simulink model "LSTM_Acc"  (R2024b)
settings: Solver=FixedStepDiscrete  StartTime=0.0  StopTime=10.0  RelTol=1e-3
libraries: rtlinux_Library x11, simulink x2, deeplib x1
settings Model: Creator=petrc  LastModifiedBy=petrc
settings OptimizationCC: DefaultParameterBehavior=Inlined  EnhancedBackFolding=on  PassReuseOutputArgsAs=Individual arguments  ZeroExternalMemoryAtStartup=off  ZeroInternalMemoryAtStartup=off  OptimizeBlockOrder=speed  DifferentSizesBufferReuse=on  OptimizationCustomize=off  EfficientTunableParamExpr=on
settings DebuggingCC: ParameterTunabilityLossMsg=error
settings HardwareCC: ProdBitPerLong=64  ProdLargestAtomicInteger=LongLong  ProdLargestAtomicFloat=Double  ProdLongLongMode=on  ProdHWDeviceType=ARM Compatible->ARM Cortex-A (64-bit)
settings SFSimCC: MATLABDynamicMemAlloc=off
settings RTWCC: Description=Real-Time Linux (WSL/Yocto)  SystemTargetFile=rtlinux_ert.tlc  MakeCommand=make_rtw \  GenerateMakefile=off  TemplateMakefile=rtlinux_ert.tmf
settings CodeAppCC: ForceParamTrailComments=on  IgnoreCustomStorageClasses=off  OperatorAnnotations=on  SimulinkDataObjDesc=on  SFDataObjDesc=on  InsertBlockDesc=on
settings STFCustomTargetCC: TargetLibSuffix=.a  TargetLangStandard=C99 (ISO)  MultiwordLength=256  GenerateSampleERTMain=on  CombineOutputUpdateFcns=on  ERTCustomFileBanners=on  SupportContinuousTime=off  SupportNonInlinedSFcns=off  RemoveResetFunc=on  MATLABClassNameForMDSCustomization=Simulink.SoftwareTarget.ERTCustomization  ModelStepFunctionPrototypeControlCompliant=on  SystemTargetFile=rtlinux_ert.tlc
settings ERTTargetCC: TargetLangStandard=C99 (ISO)  GenerateSampleERTMain=on  ParMdlRefBuildCompliant=off  CompOptLevelCompliant=off  ConcurrentExecutionCompliant=off  CPPClassGenCompliant=off  UseToolchainInfoCompliant=off  ERTCustomFileTemplate=rtlinux_file_process.tlc

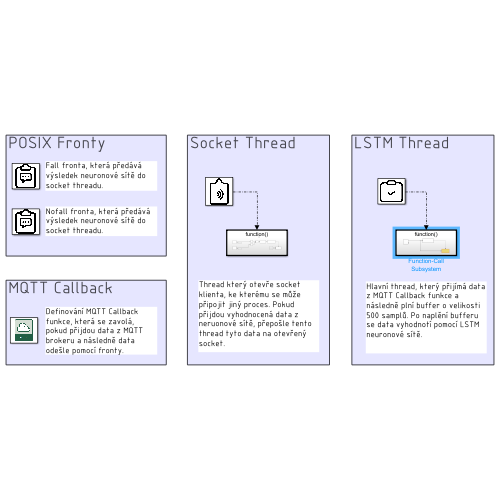
[thumbnail: Simulink's stored preview of the top-level diagram]
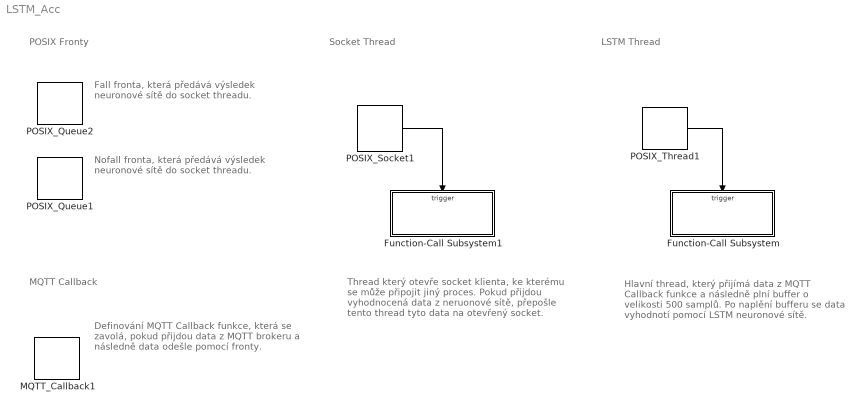
== system LSTM_Acc ==
  note: Nofall fronta, která předává výsledek neuronové sítě do socket threadu.
  note: Definování MQTT Callback funkce, která se zavolá, pokud přijdou data z MQTT brokeru a následně data odešle pomocí fronty.
  note: Socket Thread
  note: Thread který otevře socket klienta, ke kterému se může připojit jiný proces. Pokud přijdou vyhodnocená data z neruonové sítě, přepošle tento thread tyto data na otevřený socket.
  note: Fall fronta, která předává výsledek neuronové sítě do socket threadu.
  note: POSIX Fronty
  note: LSTM Thread
  note: Hlavní thread, který přijímá data z MQTT Callback funkce a následně plní buffer o velikosti 500 samplů. Po naplění bufferu se data vyhodnotí pomocí LSTM neuronové sítě.
  note: MQTT Callback
  Function-Call Subsystem : Subsystem  TreatAsAtomicUnit=on
  Function-Call Subsystem1 : Subsystem  TreatAsAtomicUnit=on
  MQTT_Callback1 : rtlinux_Library/MQTT_Callback  address=tcp://192.168.0.117:1883  clientid=CSubscriber  topic=/mpu6050/accel  qos=1  data_n=1  queue_name=accel_queue  length=10
      settings: SourceProductName=LINUX Library
  POSIX_Queue1 : rtlinux_Library/POSIX_Queue  QueueName=nofall_queue  QueueLenght=5
      settings: SourceProductName=LINUX Library
  POSIX_Queue2 : rtlinux_Library/POSIX_Queue  QueueName=fall_queue  QueueLenght=5
      settings: SourceProductName=LINUX Library
  POSIX_Socket1 : rtlinux_Library/POSIX_Socket  SocketName=/tmp/mysocket  Backlog=5  tickRes=10
      settings: SourceProductName=LINUX Library
  POSIX_Thread1 : rtlinux_Library/POSIX_Thread  TaskName=lstm_thread  TickRes=10  SchedPolicy=SCHED_OTHER  ThreadPriority=0  LockMemory=on  Affinity0=on  Affinity1=on  Affinity2=on  Affinity3=on
      settings: SourceProductName=LINUX Library
  wires:
  POSIX_Thread1/1 -> Function-Call Subsystem/Trigger
  POSIX_Socket1/1 -> Function-Call Subsystem1/Trigger

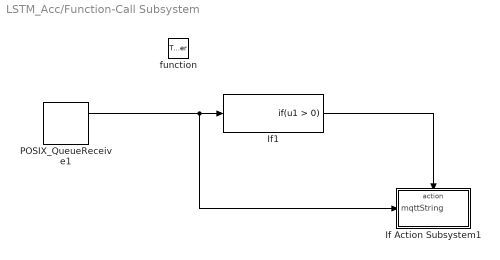
== system LSTM_Acc/Function-Call Subsystem ==
  function : TriggerPort  TriggerType=function-call  VariantControl=(inherit)
  If Action Subsystem1 : Subsystem  TreatAsAtomicUnit=on
  If1 : If  ShowElse=off
  POSIX_QueueReceive1 : rtlinux_Library/POSIX_QueueReceive  QueueName=accel_queue  buffer_enable=1  buffer_size=1024  buffer_name=receive_buffer
      settings: SourceProductName=LINUX Library
  wires:
  If1/1 -> If Action Subsystem1/Action
  POSIX_QueueReceive1/1 -> If Action Subsystem1/1(mqttString), If1/1

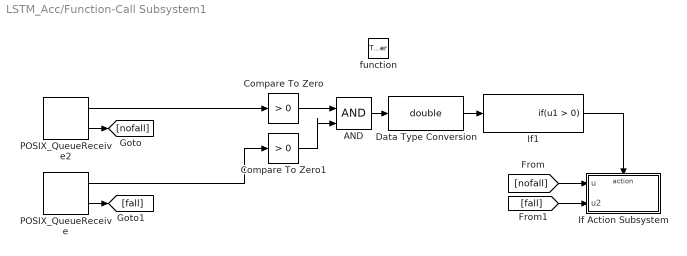
== system LSTM_Acc/Function-Call Subsystem1 ==
  function : TriggerPort  TriggerType=function-call  VariantControl=(inherit)
  AND : Logic  IconShape=distinctive  AllPortsSameDT=off  OutDataTypeStr=boolean
  Compare To Zero : simulink/Logic and Bit Operations/Compare To Zero  relop=>  OutDataTypeStr=boolean
  Compare To Zero1 : simulink/Logic and Bit Operations/Compare To Zero  relop=>  OutDataTypeStr=boolean
  Data Type Conversion : DataTypeConversion  OutDataTypeStr=double  SaturateOnIntegerOverflow=off  RndMeth=Floor
  If Action Subsystem : Subsystem  TreatAsAtomicUnit=on
  If1 : If  ShowElse=off
  POSIX_QueueReceive : rtlinux_Library/POSIX_QueueReceive  QueueName=fall_queue  buffer_enable=0  buffer_size=0  buffer_name=0
      settings: SourceProductName=LINUX Library
  POSIX_QueueReceive2 : rtlinux_Library/POSIX_QueueReceive  QueueName=nofall_queue  buffer_enable=0  buffer_size=0  buffer_name=0
      settings: SourceProductName=LINUX Library
  wires:
  POSIX_QueueReceive2/1 -> Compare To Zero/1
  POSIX_QueueReceive/1 -> Compare To Zero1/1
  If1/1 -> If Action Subsystem/Action
  POSIX_QueueReceive2/2 -> [nofall]
  POSIX_QueueReceive/2 -> [fall]
  [nofall] -> If Action Subsystem/1(u)
  [fall] -> If Action Subsystem/2(u2)
  Compare To Zero/1 -> AND/1
  Compare To Zero1/1 -> AND/2
  AND/1 -> Data Type Conversion/1
  Data Type Conversion/1 -> If1/1

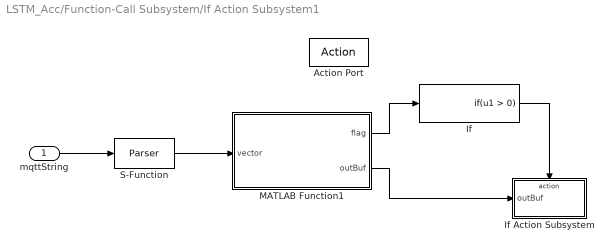
== system LSTM_Acc/Function-Call Subsystem/If Action Subsystem1 ==
  mqttString : Inport
  Action Port : ActionPort  ActionPortLabel=if(u1 > 0)
  If : If  ShowElse=off
  If Action Subsystem : Subsystem  TreatAsAtomicUnit=on
  MATLAB Function1 : MATLAB Function  TreatAsAtomicUnit=on
  S-Function : S-Function  FunctionName=Parser  SFunctionDeploymentMode=off  EnableBusSupport=off
  wires:
  If/1 -> If Action Subsystem/Action
  MATLAB Function1/1(flag) -> If/1
  MATLAB Function1/2(outBuf) -> If Action Subsystem/1(outBuf)
  mqttString/1 -> S-Function/1
  S-Function/1 -> MATLAB Function1/1(vector)

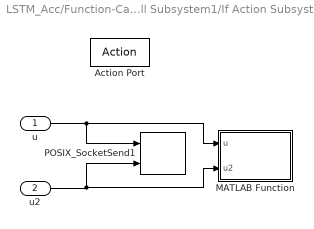
== system LSTM_Acc/Function-Call Subsystem1/If Action Subsystem ==
  u : Inport
  u2 : Inport  Port=2
  Action Port : ActionPort  ActionPortLabel=if(u1 > 0)
  MATLAB Function : MATLAB Function  TreatAsAtomicUnit=on
  POSIX_SocketSend1 : rtlinux_Library/POSIX_SocketSend  statement=%.3f %.3f  data_num=2
      settings: SourceProductName=LINUX Library
  wires:
  u/1 -> POSIX_SocketSend1/1, MATLAB Function/1(u)
  u2/1 -> POSIX_SocketSend1/2, MATLAB Function/2(u2)

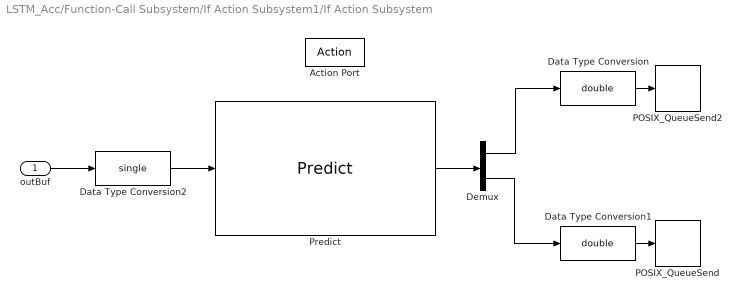
== system LSTM_Acc/Function-Call Subsystem/If Action Subsystem1/If Action Subsystem ==
  outBuf : Inport
  Action Port : ActionPort  ActionPortLabel=if(u1 > 0)
  Data Type Conversion : DataTypeConversion  OutDataTypeStr=double  SaturateOnIntegerOverflow=off  RndMeth=Floor
  Data Type Conversion1 : DataTypeConversion  OutDataTypeStr=double  SaturateOnIntegerOverflow=off  RndMeth=Floor
  Data Type Conversion2 : DataTypeConversion  OutDataTypeStr=single  SaturateOnIntegerOverflow=off  RndMeth=Floor
  Demux : Demux  Outputs=2
  POSIX_QueueSend : rtlinux_Library/POSIX_QueueSend  QueueName=fall_queue
      settings: SourceProductName=LINUX Library
  POSIX_QueueSend2 : rtlinux_Library/POSIX_QueueSend  QueueName=nofall_queue
      settings: SourceProductName=LINUX Library
  Predict : deeplib/Predict  Network=Network from MAT-file  NetworkFunction=squeezenet  NetworkFilePath=C:\Users\petrc\MATLAB\rtlinux_ert\Examples\LSTM_Acc\net.mat  MiniBatchSize=128  InputDataFormats={'sequenceinput', 'TCB';}  Predictions=on  Activations={}  ForceInterpretedSim=off  EnableDLNetwork=on  LastKnownNetworkFilePath='C:\Users\petrc\MATLAB\rtlinux_ert\Examples\LSTM_Acc\net.mat'  LastKnownNetworkTimeStamp=739733.731168981525115668773651123046875
  wires:
  Demux/1 -> Data Type Conversion/1
  Demux/2 -> Data Type Conversion1/1
  Data Type Conversion/1 -> POSIX_QueueSend2/1
  Data Type Conversion1/1 -> POSIX_QueueSend/1
  Predict/1 -> Demux/1
  Data Type Conversion2/1 -> Predict/1
  outBuf/1 -> Data Type Conversion2/1

== matlab function LSTM_Acc/Function-Call Subsystem1/If Action Subsystem/MATLAB Function ==
  data: u input; u2 input
function fcn(u, u2)

fprintf("Output: %f, %f\n\r", u, u2);

== matlab function LSTM_Acc/Function-Call Subsystem/If Action Subsystem1/MATLAB Function1 ==
  data: flag output; vector input double size=30; outBuf output
function [flag, outBuf] = buffer(vector)

persistent buf count
if isempty(buf)
    buf = zeros(500, 3);
    count = 0;
end

for i = 1:3:30
    count = count + 1;
    if count <= 500
        buf(count, :) = vector(i:i+2);
    end
end

% Check if full
if count == 500
    outBuf = buf;
    flag = 1;
    count = 0;
else
    outBuf = zeros(500, 3);
    flag = 0;
end
